simulink model "motor"  (R2021a)
settings: Solver=ode23tb  StartTime=0.0  StopTime=6  RelTol=1e-3  EnableMultiTasking=on
undefined symbols (not defined in the file): D1, lagging, pulse
libraries: spsDCMachineLib x1, spsDCVoltageSourceLib x1, spsPLL3phLib x1, spsPulseGeneratorThyristor12PulseLib x1, spsParallelRLCBranchLib x1, spsThreePhaseVIMeasurementLib x1, spsThreePhaseSourceLib x1, spsVoltageMeasurementLib x1, spsUniversalBridgeLib x1, spspowerguiLib x1
settings Model: Creator=dingmingbo  LastModifiedBy=Fuxi Wang
settings SolverCC: AlgebraicLoopSolver=TrustRegion
settings DataIOCC: LimitDataPoints=on  SaveFormat=Array  ReturnWorkspaceOutputs=off
settings OptimizationCC: LifeSpan=inf
settings DebuggingCC: SFUnexpectedBacktrackingDiag=warning  SFNoUnconditionalDefaultTransitionDiag=warning  SFExecutionAtInitializationDiag=none  SFMachineParentedDataDiag=warning  ArithmeticOperatorsInVariantConditions=warning
settings HardwareCC: ProdBitPerLong=64  ProdLargestAtomicFloat=None  ProdLongLongMode=on  ProdHWDeviceType=Generic->64-bit Embedded Processor (LP64)  TargetBitPerLong=64  TargetBitPerPointer=64  TargetLongLongMode=on  TargetWordSize=64  TargetHWDeviceType=Generic->64-bit Embedded Processor (LP64)
settings ModelReferenceCC: PropagateSignalLabelsOutOfModel=off
settings SFSimCC: SimUseLocalCustomCode=off  CustomCodeUndefinedFunction=UseInterfaceOnly
settings RTWCC: RTWUseLocalCustomCode=off
settings CodeAppCC: StateflowObjectComments=on
settings GRTTargetCC: TargetLangStandard=C89/C90 (ANSI)
settings ConfigComp: CovMetricSettings=dw  CovSaveCumulativeToWorkspaceVar=on  CovSaveSingleToWorkspaceVar=on  CovExternalEMLEnable=off
settings SimscapeCC: SimscapeNormalizeSystem=off

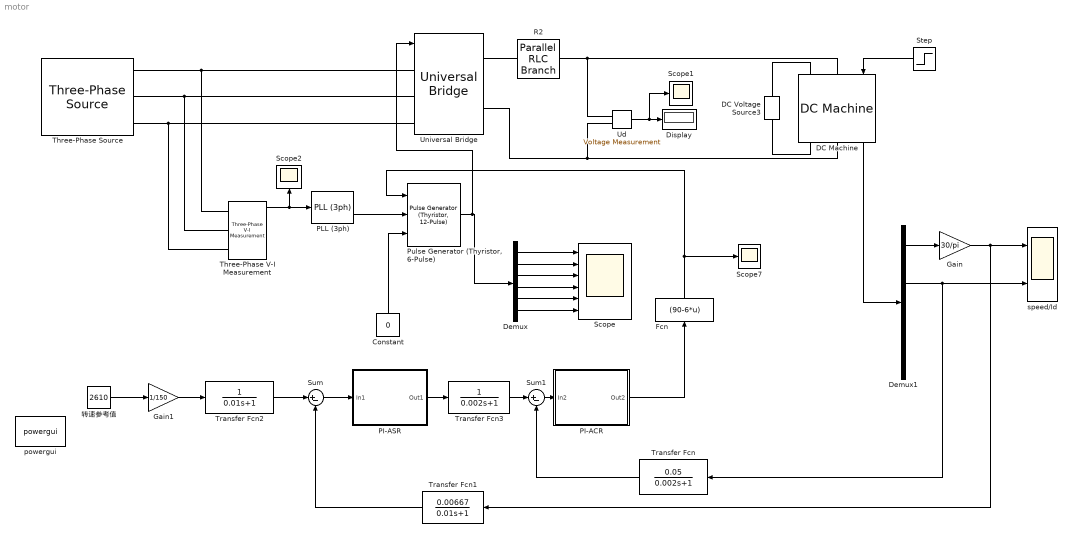
== system motor ==
  Constant : Constant  Value=0
  DC Machine : spsDCMachineLib/DC Machine  PresetModel=No  MechanicalLoad=Torque TL  FieldType=Wound  ShowDetailedParameters=on  MeasurementBus=off  RLa="[0.368  0.00021]"  RLf="[ 146.7  0]"  Laf=0.84  MachineConstant=Torque constant (N.m/A)  Ke=1.8  Kt=1.8  J=0.57  Bm=0  Tf=0  w0=1  Ifinit=1  TsPowergui=0  TsBlock=-1
  DC Voltage Source3 : spsDCVoltageSourceLib/DC Voltage Source  Amplitude=220  Measurements=None
  Demux : Demux  Outputs=6
  Demux1 : Demux
  Display : Display
  Fcn : Fcn  Expr=(90-6*u)
  Gain : Gain  Gain=30/pi
  Gain1 : Gain  Gain=1/150
  PI-ACR : Subsystem
  PI-ASR : Subsystem
  PLL (3ph) : spsPLL3phLib/PLL (3ph)  Fmin=45  Par_Init=[0, 50]  ParK=[180, 3200, 1]  TcD=1e-4  MaxRateChangeFreq=12  FilterCutOffFreq=25  Ts=0  AGC=on
  "Pulse Generator (Thyristor, 6-Pulse)" : spsPulseGeneratorThyristor12PulseLib/Pulse Generator (Thyristor, 12-Pulse)  GenType=6-pulse  Delta=D1 (lagging)  pwidth=50  Double_Pulse=off  Ts=0
      settings: SourceProductBaseCode=PS
  R2 : spsParallelRLCBranchLib/Parallel RLC Branch  LConnTagsString=a  RConnTagsString=__new0  BranchType=L  Resistance=0.1  Inductance=0.02  SetiL0=off  InitialCurrent=0  Capacitance=1  Setx0=off  InitialVoltage=0  Measurements=None
  Scope : Scope  NumInputPorts=6
  Scope1 : Scope
  Scope2 : Scope
  Scope7 : Scope
  Step : Step  Time=0  After=171.4  SampleTime=0
  Sum : Sum  Inputs=|+-
  Sum1 : Sum  Inputs=|+-
  Three-Phase V-I Measurement : spsThreePhaseVIMeasurementLib/Three-Phase V-I Measurement  VoltageMeasurement=phase-to-ground  SetLabelV=off  LabelV=Vabc  Vpu=off  VpuLL=off  CurrentMeasurement=yes  SetLabelI=off  LabelI=Iabc  Ipu=off  Pbase=100e6  Vbase=500e3  OutputType=Complex  PhasorSimulation=off  PSBequivalent=0
  Three-Phase Source : spsThreePhaseSourceLib/Three-Phase Source  InternalConnection=Yg  VoltagePhases=off  Voltage=380  PhaseAngle=0  Voltage_phases=[25e3 25e3 25e3]/sqrt(3)  PhaseAngles_phases=[0 -120 +120]  Frequency=50  NonIdealSource=on  SpecifyImpedance=off  Resistance=0  Inductance=0  ShortCircuitLevel=100e6  BaseVoltage=380  XRratio=7  BusType=swing  Pref=10e3  Qref=0  Prefabc=[10e3, 10e3, 10e3]  Qrefabc=[0, 0, 0]  Qmin=-inf  Qmax=inf
  Transfer Fcn : TransferFcn  Numerator=[0.05]  Denominator=[0.002 1]
  Transfer Fcn1 : TransferFcn  Numerator=[0.00667]  Denominator=[0.01 1]
  Transfer Fcn2 : TransferFcn  Denominator=[0.01 1]
  Transfer Fcn3 : TransferFcn  Denominator=[0.002 1]
  Ud : spsVoltageMeasurementLib/Voltage Measurement  PhasorSimulation=off  OutputType=Complex  PSBequivalent=0
  Universal Bridge : spsUniversalBridgeLib/Universal Bridge  Arms=3  SnubberResistance=1e5  SnubberCapacitance=inf  Device=Thyristors  Ron=1e-3  Lon=0  ForwardVoltages="[  0  0  ]"  ForwardVoltage=0  GTOparameters=[ 10e-6 , 20e-6 ]  IGBTparameters=[ 1e-6 , 2e-6 ]  Measurements=None  Measurements_2=None  converterType=Rectifier
  powergui : spspowerguiLib/powergui  Priority=1  SimulationMode=Continuous  SampleTime=50e-6  frequency=60  Iterations=50  frequencyindice=0  Pbase=100e6  ErrMax=1e-4  UnitsV=kV  UnitsW=MW  buscounter=0  FunctionMessages=off  echomessages=off  EnableUseOfTLC=off  CurrentSourceSwitches=on  DisableSnubberDevices=off  DisableRonSwitches=off  DisableVfSwitches=off  DisplayEquations=off  AutomaticDiscreteSolvers=off  SolverType=Tustin/Backward Euler (TBE)  Interpol=off  ExternalGateDelay=off  methode=off  Ts=100  x0status=blocks  SPID=off  SwTol=0  HookPort=off  NonlinearTolerance=1e-4  nMaxIteration=100  ContinueOnMaxIteration=off  RestoreLinks=warning  ResistiveCurrentMeasurement=off  Frange=[0:2:500]  Ylog=off  Xlog=on  ShowGrid=off  save=off  variable=ZData  structure=0  ZoomFFT=off  StartTime=0.0  cycles=1  DisplayStyle=1  fundamental=60  FreqAxis=off  MaxFrequency=1000  frequencyindicesteady=1  RmsSteady=1  display=off
  speed/Id : Scope  NumInputPorts=2
  转速参考值 : Constant  Value=2610
  wires:
  Three-Phase V-I Measurement/1 -> PLL (3ph)/1, Scope2/1
  PLL (3ph)/2 -> "Pulse Generator (Thyristor, 6-Pulse)"/2
  Constant/1 -> "Pulse Generator (Thyristor, 6-Pulse)"/3
  "Pulse Generator (Thyristor, 6-Pulse)"/1 -> Universal Bridge/1, Demux/1
  Ud/1 -> Scope1/1, Display/1
  Demux/1 -> Scope/1
  Demux/2 -> Scope/2
  Demux/3 -> Scope/3
  Demux/5 -> Scope/5
  Demux/4 -> Scope/4
  Demux/6 -> Scope/6
  DC Machine/1 -> Demux1/1
  Demux1/1 -> Gain/1
  Gain/1 -> Transfer Fcn1/1, speed/Id/1
  Demux1/2 -> speed/Id/2, Transfer Fcn/1
  Step/1 -> DC Machine/1
  Transfer Fcn1/1 -> Sum/2
  Transfer Fcn2/1 -> Sum/1
  Sum/1 -> PI-ASR/1(In1)
  PI-ASR/1(Out1) -> Transfer Fcn3/1
  Transfer Fcn3/1 -> Sum1/1
  Transfer Fcn/1 -> Sum1/2
  Sum1/1 -> PI-ACR/1(In2)
  转速参考值/1 -> Gain1/1
  Gain1/1 -> Transfer Fcn2/1
  PI-ACR/1(Out2) -> Fcn/1
  Fcn/1 -> Scope7/1, "Pulse Generator (Thyristor, 6-Pulse)"/1
  connections:
  Three-Phase V-I Measurement/LConn1 -- Three-Phase Source/RConn1 -- Universal Bridge/LConn1
  Three-Phase Source/RConn2 -- Universal Bridge/LConn2 -- Three-Phase V-I Measurement/LConn2
  Three-Phase Source/RConn3 -- Universal Bridge/LConn3 -- Three-Phase V-I Measurement/LConn3
  DC Machine/LConn1 -- R2/LConn1 -- Ud/LConn1
  Ud/LConn2 -- Universal Bridge/RConn2 -- DC Machine/RConn1
  DC Voltage Source3/LConn1 -- DC Machine/RConn2
  DC Voltage Source3/RConn1 -- DC Machine/LConn2
  Universal Bridge/RConn1 -- R2/RConn1

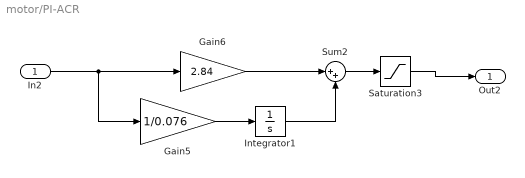
== system motor/PI-ACR ==
  In2 : Inport
  Gain5 : Gain  Gain=1/0.076
  Gain6 : Gain  Gain=2.84
  Integrator1 : Integrator  LimitOutput=on  UpperSaturationLimit=12  LowerSaturationLimit=-12
  Saturation3 : Saturate  UpperLimit=10  LowerLimit=-10
  Sum2 : Sum  Inputs=|++
  Out2 : Outport  VectorParamsAs1DForOutWhenUnconnected=off
  wires:
  Sum2/1 -> Saturation3/1
  Gain5/1 -> Integrator1/1
  Gain6/1 -> Sum2/1
  Integrator1/1 -> Sum2/2
  In2/1 -> Gain5/1, Gain6/1
  Saturation3/1 -> Out2/1

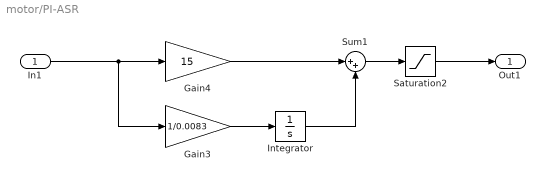
== system motor/PI-ASR ==
  In1 : Inport
  Gain3 : Gain  Gain=1/0.0083
  Gain4 : Gain  Gain=15
  Integrator : Integrator  LimitOutput=on  UpperSaturationLimit=12  LowerSaturationLimit=-12
  Saturation2 : Saturate  UpperLimit=10  LowerLimit=-10
  Sum1 : Sum  Inputs=|++
  Out1 : Outport  VectorParamsAs1DForOutWhenUnconnected=off
  wires:
  Sum1/1 -> Saturation2/1
  Saturation2/1 -> Out1/1
  Integrator/1 -> Sum1/2
  In1/1 -> Gain3/1, Gain4/1
  Gain3/1 -> Integrator/1
  Gain4/1 -> Sum1/1
